simulink model "Model"  (R2021a)
settings: Solver=VariableStepAuto  StartTime=0.0  StopTime=20  MaxStep=0.005  RelTol=1e-5
values from neighbouring files (symbols this model uses):
  b = 12.5    [invertedPendulumInit.m]
  d = 0.0019    [invertedPendulumInit.m]
  friction_coefficient = (deadzone * v_supply_max/r_pulley/Ra/pwm_max)    (= 91.0580950647)    [invertedPendulumInit.m]
  g = 9.81    [invertedPendulumInit.m]
  K = lqr(A,B,Q,R)    [invertedPendulumInit.m]
  K_pwm = v_supply_max*Kt/r_pulley/Ra/pwm_max/N    (= 0.143180319444)    [invertedPendulumInit.m]
  Kt = 0.141516564131871    (= 0.141516564132)    [invertedPendulumInit.m]
  l = 0.5    [invertedPendulumInit.m]
  M = 1.1571    [invertedPendulumInit.m]
  m = 0.3    [invertedPendulumInit.m]
  x = 3    [invertedPendulumInit.m]
undefined symbols (not defined in the file or in its folder): DiscIntNeverNeededParam
libraries: simulink_extras x1, dspsigops x1
settings Model: Creator=extra  LastModifiedBy=2000r
settings SolverCC: AlgebraicLoopSolver=TrustRegion
settings DataIOCC: InspectSignalLogs=on  ReturnWorkspaceOutputsName=SDOSimTest_Log
settings DebuggingCC: SFMachineParentedDataDiag=warning

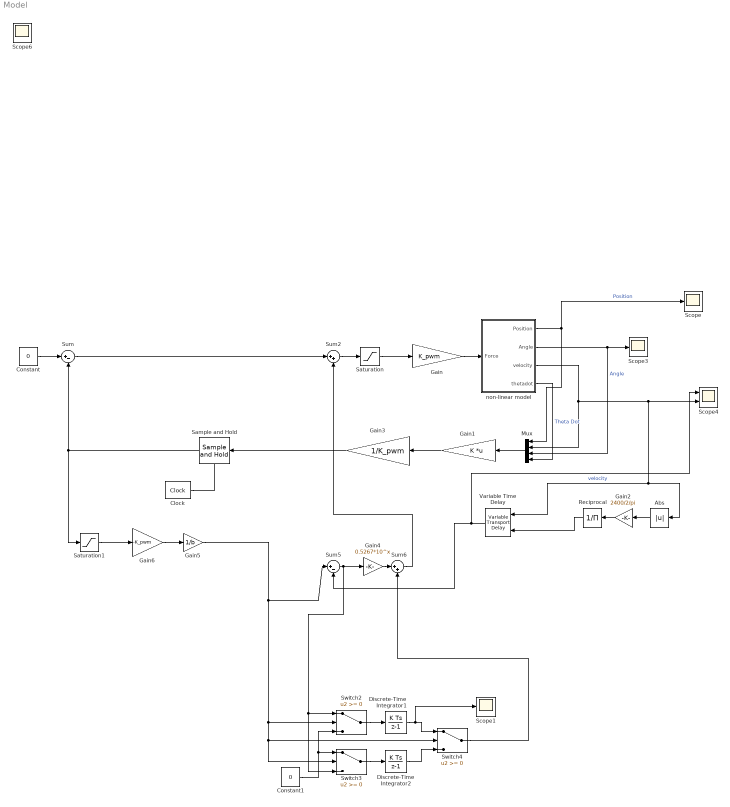
== system Model ==
  Abs : Abs
  Clock : simulink_extras/Flip Flops/Clock  period=0.005
  Constant : Constant  Value=0
  Constant1 : Constant  Value=0
  Discrete-Time Integrator1 : DiscreteIntegrator  gainval=5.498*10^x  SampleTime=0.005  LimitOutput=on  UpperSaturationLimit=50  LowerSaturationLimit=-50  ICPrevOutput=DiscIntNeverNeededParam  ICPrevScaledInput=DiscIntNeverNeededParam
  Discrete-Time Integrator2 : DiscreteIntegrator  gainval=5.498*10^x  SampleTime=0.005  LimitOutput=on  UpperSaturationLimit=50  LowerSaturationLimit=-50  ICPrevOutput=DiscIntNeverNeededParam  ICPrevScaledInput=DiscIntNeverNeededParam
  Gain : Gain  Gain=K_pwm
  Gain1 : Gain  Gain=K  Multiplication=Matrix(K*u)
  Gain2 : Gain  Gain=2400/2/pi
  Gain3 : Gain  Gain=1/K_pwm
  Gain4 : Gain  Gain=0.5267*10^x
  Gain5 : Gain  Gain=1/b
  Gain6 : Gain  Gain=-K_pwm
  Mux : Mux
  Reciprocal : Product  Inputs=/
  Sample and Hold : dspsigops/Sample and Hold  trig=Rising edge  initCond=0  latchinput=off
  Saturation : Saturate  UpperLimit=255  LowerLimit=-255
  Saturation1 : Saturate  UpperLimit=255  LowerLimit=-255
  Scope{,1,3,6} (4 alike) : Scope
  Scope4 : Scope  NumInputPorts=2
  Sum : Sum  Inputs=|+-
  Sum2 : Sum  Inputs=|++
  Sum5 : Sum  Inputs=|+-
  Sum6 : Sum  Inputs=|++
  Switch2 : Switch  ZeroCross=off
  Switch3 : Switch  ZeroCross=off
  Switch4 : Switch  ZeroCross=off
  Variable Time Delay : VariableTransportDelay  VariableDelayType=Variable transport delay  MaximumDelay=0.2
  non-linear model : Subsystem
  wires:
  Gain/1 -> non-linear model/1(Force)
  Clock/1 -> Sample and Hold/Trigger
  Gain6/1 -> Gain5/1
  Sample and Hold/1 -> Saturation1/1, Sum/2
  Gain1/1 -> Gain3/1
  Sum/1 -> Sum2/1
  Constant/1 -> Sum/1
  Saturation1/1 -> Gain6/1
  Sum2/1 -> Saturation/1
  Gain3/1 -> Sample and Hold/1
  Saturation/1 -> Gain/1
  non-linear model/1(Position) -> Scope/1, Mux/1  "Position"
  Mux/1 -> Gain1/1
  non-linear model/4(thetadot) -> Mux/4  "Theta Dot"
  non-linear model/2(Angle) -> Scope3/1, Mux/3  "Angle"
  Gain2/1 -> Reciprocal/1
  Reciprocal/1 -> Variable Time Delay/2
  non-linear model/3(velocity) -> Scope4/2, Variable Time Delay/1, Abs/1, Mux/2  "velocity"
  Abs/1 -> Gain2/1
  Switch4/1 -> Sum6/2
  Switch3/1 -> Discrete-Time Integrator2/1
  Constant1/1 -> Switch3/1, Switch2/3
  Gain5/1 -> Switch4/2, Switch3/2, Switch2/2, Sum5/1
  Gain4/1 -> Sum6/1
  Discrete-Time Integrator2/1 -> Switch4/3
  Switch2/1 -> Discrete-Time Integrator1/1
  Discrete-Time Integrator1/1 -> Scope1/1, Switch4/1
  Variable Time Delay/1 -> Sum5/2, Scope4/1
  Sum5/1 -> Switch3/3, Switch2/1, Gain4/1
  Sum6/1 -> Sum2/2

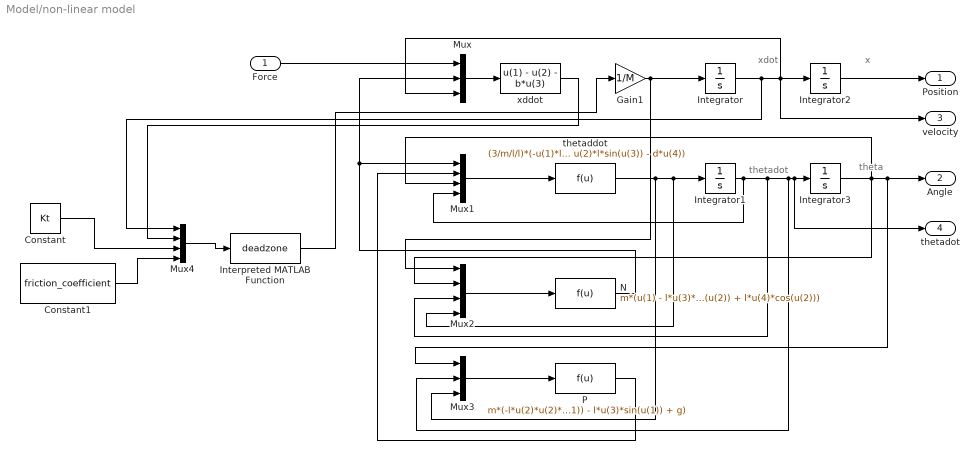
== system Model/non-linear model ==
  note: theta
  note: thetadot
  note: xdot
  note: x
  Force : Inport
  Constant : Constant  Value=Kt
  Constant1 : Constant  Value=friction_coefficient
  Gain1 : Gain  Gain=1/M
  Integrator : Integrator  ContinuousStateAttributes='xdot'
  Integrator1 : Integrator  ContinuousStateAttributes='thetadot'
  Integrator2 : Integrator  ContinuousStateAttributes='x'
  Integrator3 : Integrator  InitialCondition=0.17  ContinuousStateAttributes='theta'
  Interpreted MATLAB Function : MATLABFcn  MATLABFcn=deadzone
  Mux : Mux  Inputs=3
  Mux1 : Mux
  Mux2 : Mux
  Mux3 : Mux  Inputs=3
  Mux4 : Mux
  N : Fcn  Expr=m*(u(1) - l*u(3)*u(3)*sin(u(2)) + l*u(4)*cos(u(2)))
  P : Fcn  Expr=m*(-l*u(2)*u(2)*cos(u(1)) - l*u(3)*sin(u(1)) + g)
  thetaddot : Fcn  Expr=(3/m/l/l)*(-u(1)*l*cos(u(3)) + u(2)*l*sin(u(3)) - d*u(4))
  xddot : Fcn  Expr=u(1) - u(2) - b*u(3)
  Position : Outport
  Angle : Outport  Port=2
  velocity : Outport  Port=3
  thetadot : Outport  Port=4
  wires:
  thetaddot/1 -> Mux3/3, Mux2/4, Integrator1/1
  Mux4/1 -> Interpreted MATLAB Function/1
  Mux/1 -> xddot/1
  Constant/1 -> Mux4/3
  Mux1/1 -> thetaddot/1
  Interpreted MATLAB Function/1 -> Gain1/1
  Integrator3/1 -> Mux2/2, Mux1/3, Angle/1, Mux3/1
  P/1 -> Mux1/2
  Integrator1/1 -> Mux1/4, Mux2/3, Mux3/2, thetadot/1, Integrator3/1
  Integrator/1 -> Mux4/1, velocity/1, Mux/3, Integrator2/1
  Gain1/1 -> Mux2/1, Integrator/1
  N/1 -> Mux1/1, Mux/2
  Mux3/1 -> P/1
  Mux2/1 -> N/1
  Force/1 -> Mux/1
  xddot/1 -> Mux4/2
  Integrator2/1 -> Position/1
  Constant1/1 -> Mux4/4
